simulink model "AltitudeControl"  (R2017b)
settings: Solver=FixedStepDiscrete  StartTime=0.0  StopTime=100.0  FixedStep=2.000000  RelTol=1e-3
undefined symbols (not defined in the file): DiscIntNeverNeededParam
settings Model: Creator=hbourbou  LastModifiedBy=hbourbou
settings OptimizationCC: LifeSpan=inf
settings DebuggingCC: SFExecutionAtInitializationDiag=none
settings HardwareCC: ProdBitPerSizeT=32  ProdBitPerPtrDiffT=32  ProdWordSize=32  ProdHWDeviceType=Specified
settings CodeAppCC: StateflowObjectComments=on

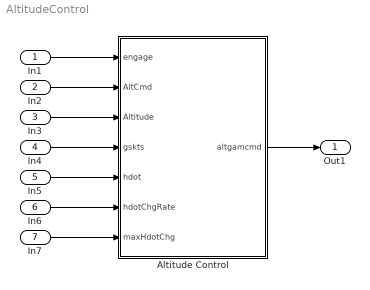
== system AltitudeControl ==
  In1 : Inport
  In2 : Inport  Port=2
  In3 : Inport  Port=3
  In4 : Inport  Port=4
  In5 : Inport  Port=5
  In6 : Inport  Port=6
  In7 : Inport  Port=7
  Altitude Control : Subsystem  RequirementInfo={'other' '..\..\tcm_requirements.docx' '@Simulink_requirement_item_14' 'true' 'Altitude Control' '' } %GIDa_d6bc4744_614c_4bb5_9453_e66fb0200636
  Out1 : Outport
  wires:
  In1/1 -> Altitude Control/1(engage)
  In2/1 -> Altitude Control/2(AltCmd)
  In3/1 -> Altitude Control/3(Altitude)
  In4/1 -> Altitude Control/4(gskts)
  In5/1 -> Altitude Control/5(hdot)
  In6/1 -> Altitude Control/6(hdotChgRate)
  In7/1 -> Altitude Control/7(maxHdotChg)
  Altitude Control/1(altgamcmd) -> Out1/1

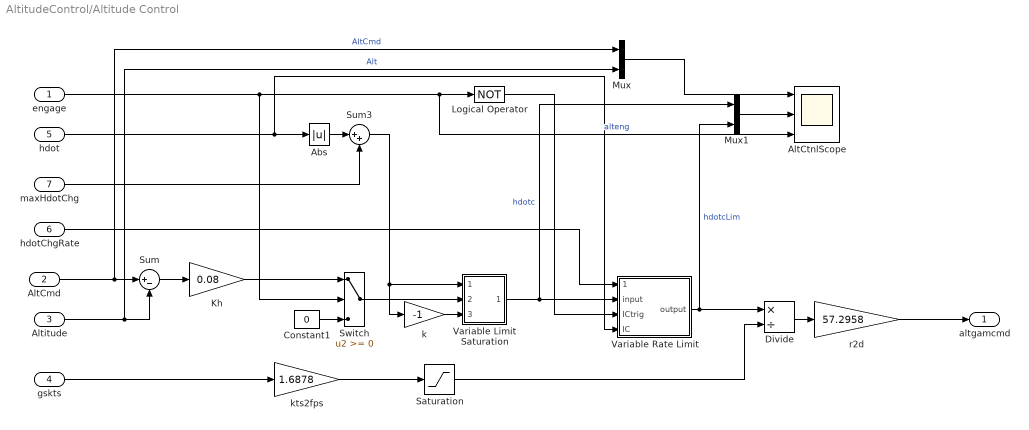
== system AltitudeControl/Altitude Control ==
  engage : Inport  RequirementInfo={} %GIDa_a0f9e7bc_5f4c_47b4_a82d_c8f7fdf97036
  AltCmd : Inport  RequirementInfo={} %GIDa_d1dee97b_de5a_4e52_b2ce_0b485c8aa484  Port=2
  Altitude : Inport  RequirementInfo={} %GIDa_78168f54_e8d5_4756_811f_19199969968a  Port=3
  gskts : Inport  RequirementInfo={} %GIDa_ccc588d0_c685_49d6_bf9c_90b171981b1a  Port=4
  hdot : Inport  RequirementInfo={} %GIDa_9911ab89_dbf4_4035_af32_728763ac766c  Port=5
  hdotChgRate : Inport  Port=6
  maxHdotChg : Inport  Port=7
  Abs : Abs  RequirementInfo={} %GIDa_024fb668_e813_4a78_abf2_704ed43c4ce5  SaturateOnIntegerOverflow=on
  AltCtnlScope : Scope  NumInputPorts=3
      settings: RequirementInfo={} %GIDa_7e9941b0_d100_47ea_9672_99fe76181463
  Constant1 : Constant  RequirementInfo={} %GIDa_99d502bf_95c3_41c5_9d9c_fc5e1253e4b1  Value=0
  Divide : Product  RequirementInfo={} %GIDa_c868b75e_df59_475c_97f0_b3865f567906  Inputs=*/
  Kh : Gain  RequirementInfo={} %GIDa_ce754ae8_662f_4a1f_a357_55d64e16e51b  Gain=0.08
  Logical Operator : Logic  RequirementInfo={} %GIDa_9ca47fc7_64f9_49de_9202_f4d238c96326  Operator=NOT
  Mux : Mux  RequirementInfo={} %GIDa_c2fbbd77_f84e_4ec9_bebc_b8c7fa776f94  Inputs=2
  Mux1 : Mux  RequirementInfo={} %GIDa_3c4cf235_29a4_489e_81c9_eaa733a25532  Inputs=2
  Saturation : Saturate  RequirementInfo={} %GIDa_684bf5f1_32b7_4ecf_9aa0_49eb7a6b1391  UpperLimit=1000  LowerLimit=0.0001
  Sum : Sum  RequirementInfo={} %GIDa_c8c4b0ab_2620_4340_80ec_50f8885fa08e  Inputs=|+-
  Sum3 : Sum  RequirementInfo={} %GIDa_124b334f_9ff9_49cc_9e2c_9c7cae593fda  Inputs=|++  SaturateOnIntegerOverflow=on  InputSameDT=on  OutDataTypeStr=Inherit: Same as first input
  Switch : Switch  RequirementInfo={} %GIDa_50c81ca4_92f9_449b_9c60_e7687784d5cc
  Variable Rate Limit : Subsystem  RequirementInfo={} %GIDa_9ad050e7_81cb_4471_a6c9_6c0865df2d82
  Variable Limit Saturation : Subsystem  RequirementInfo={} %GIDa_92c0e65b_7aa3_4146_a1ea_81983b91745d
  k : Gain  RequirementInfo={} %GIDa_93b7c979_e207_485c_936d_f501186e1da8  Gain=-1
  kts2fps : Gain  RequirementInfo={} %GIDa_4e349b4d_e2f2_4dd0_a1dd_d38f153bf0d9  Gain=1.6878
  r2d : Gain  RequirementInfo={} %GIDa_3fd0c214_217b_45da_a2b9_6aaa443cf70d  Gain=57.2958
  altgamcmd : Outport  RequirementInfo={} %GIDa_3bb5304f_2af1_4643_b8d3_b507666af521
  wires:
  Sum/1 -> Kh/1
  AltCmd/1 -> Sum/1, Mux/1  "AltCmd"
  Altitude/1 -> Sum/2, Mux/2  "Alt"
  hdot/1 -> Abs/1, Variable Rate Limit/4(IC)
  Abs/1 -> Sum3/1
  maxHdotChg/1 -> Sum3/2
  k/1 -> Variable Limit Saturation/3(Lo_lim)
  Sum3/1 -> k/1, Variable Limit Saturation/1(up_lim)
  engage/1 -> Switch/2, Logical Operator/1, AltCtnlScope/3  "alteng"
  gskts/1 -> kts2fps/1
  Divide/1 -> r2d/1
  r2d/1 -> altgamcmd/1
  Logical Operator/1 -> Variable Rate Limit/3(ICtrig)
  Variable Limit Saturation/1(Out1) -> Variable Rate Limit/2(input), Mux1/1  "hdotc"
  hdotChgRate/1 -> Variable Rate Limit/1(ratelim)
  Variable Rate Limit/1(output) -> Divide/1, Mux1/2  "hdotcLim"
  kts2fps/1 -> Saturation/1
  Saturation/1 -> Divide/2
  Switch/1 -> Variable Limit Saturation/2(SigIn)
  Kh/1 -> Switch/1
  Constant1/1 -> Switch/3
  Mux/1 -> AltCtnlScope/1
  Mux1/1 -> AltCtnlScope/2

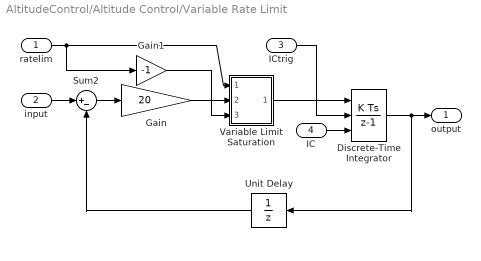
== system AltitudeControl/Altitude Control/Variable Rate Limit ==
  ratelim : Inport  RequirementInfo={} %GIDa_742cc77d_5ffc_4fb3_b8da_e15d27a45337
  input : Inport  RequirementInfo={} %GIDa_f7f634f7_100b_4972_bffd_90c72d07c499  Port=2
  ICtrig : Inport  RequirementInfo={} %GIDa_a6f5e79f_e5a9_4f54_8a40_78199250aaa7  Port=3
  IC : Inport  RequirementInfo={} %GIDa_6b8a51fb_32b8_42c7_a45b_91b406d198a8  Port=4
  Discrete-Time Integrator : DiscreteIntegrator  ExternalReset=level  InitialConditionSource=external  InitialConditionSetting=State (most efficient)  SampleTime=-1  ICPrevOutput=DiscIntNeverNeededParam  ICPrevScaledInput=DiscIntNeverNeededParam
  Gain : Gain  RequirementInfo={} %GIDa_99b7a0a4_7acf_4935_9f18_a9c4e5917a34  Gain=20  SaturateOnIntegerOverflow=on  OutDataTypeStr=Inherit: Same as input  ParamDataTypeStr=Inherit: Same as input
  Gain1 : Gain  RequirementInfo={} %GIDa_8962ac30_41c1_4429_a58b_d86829c84191  Gain=-1  SaturateOnIntegerOverflow=on  OutDataTypeStr=Inherit: Same as input  ParamDataTypeStr=Inherit: Same as input
  Sum2 : Sum  RequirementInfo={} %GIDa_8debaa47_1cfa_43e8_8c26_40a81840812b  Inputs=|+-  SaturateOnIntegerOverflow=on
  Unit Delay : UnitDelay  SampleTime=-1
  Variable Limit Saturation : Subsystem  RequirementInfo={} %GIDa_70edaf57_13d7_48dd_8e40_9c9b3e11dd41
  output : Outport  RequirementInfo={} %GIDa_5dadb99a_75f1_4cd9_8b44_3be971e9b375
  wires:
  Sum2/1 -> Gain/1
  Gain/1 -> Variable Limit Saturation/2(SigIn)
  ratelim/1 -> Gain1/1, Variable Limit Saturation/1(up_lim)
  Gain1/1 -> Variable Limit Saturation/3(Lo_lim)
  Variable Limit Saturation/1(Out1) -> Discrete-Time Integrator/1
  Discrete-Time Integrator/1 -> Unit Delay/1, output/1
  input/1 -> Sum2/1
  ICtrig/1 -> Discrete-Time Integrator/2
  IC/1 -> Discrete-Time Integrator/3
  Unit Delay/1 -> Sum2/2

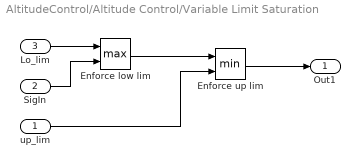
== system AltitudeControl/Altitude Control/Variable Limit Saturation ==
  up_lim : Inport  RequirementInfo={} %GIDa_e18b9e60_8b2a_44ae_b8ed_e818c73ca6e4
  SigIn : Inport  RequirementInfo={} %GIDa_3ef36df2_ffd4_4299_b72b_7afbf3d67afa  Port=2
  Lo_lim : Inport  RequirementInfo={} %GIDa_da200bdc_0c29_4663_9b89_16c3b8e7d9e2  Port=3
  Enforce low lim : MinMax  RequirementInfo={} %GIDa_3bbc4d02_d609_45e1_9e77_7e883dc504dd  Function=max  Inputs=2
  Enforce up lim : MinMax  RequirementInfo={} %GIDa_b6510814_de7e_4f5e_8e4a_65a3d0660990  Inputs=2
  Out1 : Outport  RequirementInfo={} %GIDa_16eed47c_b386_483a_84c3_b3b8fc69318d
  wires:
  Lo_lim/1 -> Enforce low lim/1
  SigIn/1 -> Enforce low lim/2
  Enforce low lim/1 -> Enforce up lim/1
  up_lim/1 -> Enforce up lim/2
  Enforce up lim/1 -> Out1/1

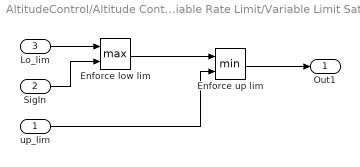
== system AltitudeControl/Altitude Control/Variable Rate Limit/Variable Limit Saturation ==
  up_lim : Inport  RequirementInfo={} %GIDa_c77d0cb4_646b_4589_b610_dbab6752c627
  SigIn : Inport  RequirementInfo={} %GIDa_a96d703e_3c86_49df_8f8d_3ed6bad87303  Port=2
  Lo_lim : Inport  RequirementInfo={} %GIDa_6165f291_f726_4a29_85c3_a12d252fc15c  Port=3
  Enforce low lim : MinMax  RequirementInfo={} %GIDa_b7d5be54_0f4d_41f1_af48_2c22347016a1  Function=max  Inputs=2
  Enforce up lim : MinMax  RequirementInfo={} %GIDa_d86a7887_eaac_49ce_9647_44f6d60ef0e9  Inputs=2
  Out1 : Outport  RequirementInfo={} %GIDa_39e435ed_73d9_4892_b6cd_765f9e1f0d00
  wires:
  Enforce up lim/1 -> Out1/1
  up_lim/1 -> Enforce up lim/2
  Enforce low lim/1 -> Enforce up lim/1
  SigIn/1 -> Enforce low lim/2
  Lo_lim/1 -> Enforce low lim/1
